simulink model "mobil_transporter"  (R2012b)
settings: Solver=FixedStepDiscrete  StartTime=0.0  StopTime=10.0  RelTol=1e-3
libraries: commutil2 x12, c2833xlib x8, c280xlib x6, idelinklib_tgtpref x2, simulink x1, idelinklib_ticcs x1
(part 1 of 2)
settings Model: Creator=User  LastModifiedBy=Gelin Wang
settings DataIOCC: SaveOutput=off  SaveTime=off
settings OptimizationCC: OptimizeModelRefInitCode=on  LifeSpan=1
settings HardwareCC: ProdBitPerChar=16  ProdBitPerInt=16  ProdBitPerPointer=16  ProdLargestAtomicInteger=Integer  ProdIntDivRoundTo=Zero  ProdEndianess=LittleEndian  ProdWordSize=16  ProdHWDeviceType=Texas Instruments->C2000
settings SFSimCC: SimCustomSourceCode="#include \"i2c_reset.c\""  SimCustomHeaderCode="#include \"i2c_reset.h\""
settings RTWCC: SystemTargetFile=idelink_ert.tlc  GenerateMakefile=off  TemplateMakefile=none  Description=IDE Link ERT  ProcessScript=idelink_ert_make_rtw_hook  RTWUseSimCustomCode=on  CustomSourceCode="#include \"i2c_reset.c\""  CustomHeaderCode="#include \"i2c_reset.h\""
settings CodeAppCC: IgnoreCustomStorageClasses=off

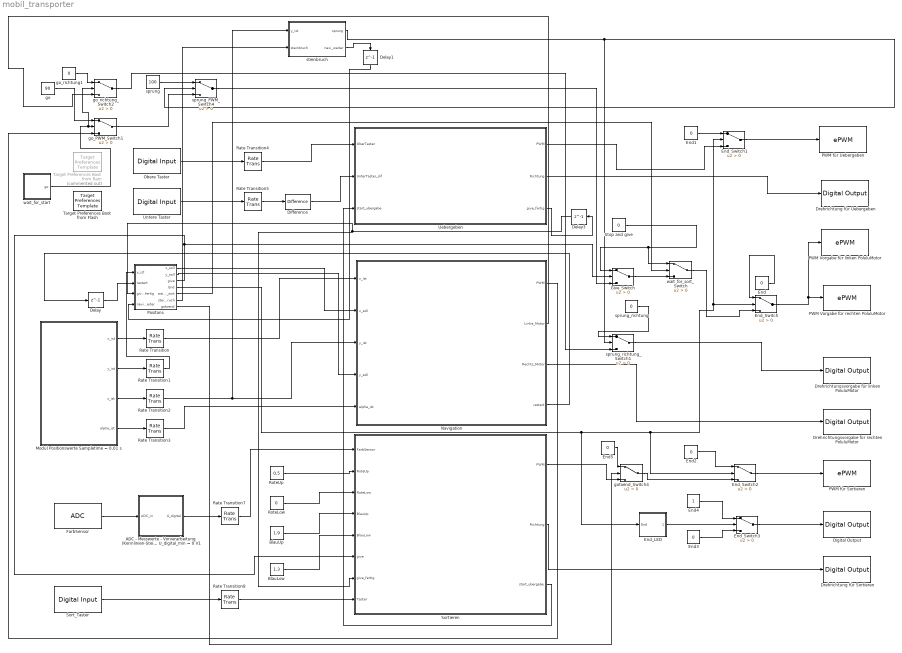
== system mobil_transporter ==
  "    go_PWM_Switch1" : Switch  Criteria=u2 > Threshold
  "    go_richtung_Switch2" : Switch  Criteria=u2 > Threshold
  "    sprung_PWM_Switch4" : Switch  Criteria=u2 > Threshold
  "    sprung_richtung_Switch1" : Switch  Criteria=u2 > Threshold
  ADC - Messwerte - Vorverarbeitung (Kennlinien-Steigung und Offset-Kompensation) U_digital = (ADC_in - Offset) * 3.546 V / 4096 mit U_digital_max = 3.546 V U_digital_min = 0 V1 : Subsystem
  BlauLow : Constant  Value=1.3
  BlauUp : Constant  Value=1.9
  Delay : Delay  DelayLength=1  InitialCondition=0
  Delay1 : Delay  DelayLength=1  InitialCondition=0
  Delay3 : Delay  DelayLength=1  InitialCondition=0
  Difference : simulink/Discrete/Difference  ICPrevInput=0.0  InputProcessing=Inherited  OutMin=[]  OutMax=[]  OutDataType=fixdt(1, 16)  OutScaling=2^-10  DoSatur=off
  Digital Output : c2833xlib/Digital Output  GPIO_Number=GPIO56~GPIO63  GPIO_Bit0=off  GPIO_BIT0_Toggle=off  GPIO_Bit1=off  GPIO_BIT1_Toggle=off  GPIO_Bit2=on  GPIO_BIT2_Toggle=off  GPIO_Bit3=off  GPIO_BIT3_Toggle=off  GPIO_Bit4=off  GPIO_BIT4_Toggle=off  GPIO_Bit5=off  GPIO_BIT5_Toggle=off  GPIO_Bit6=off  GPIO_BIT6_Toggle=off  GPIO_Bit7=off  GPIO_BIT7_Toggle=off
  Drehrichtung für Sortieren : c2833xlib/Digital Output  GPIO_Number=GPIO8~GPIO15  GPIO_Bit0=off  GPIO_BIT0_Toggle=off  GPIO_Bit1=off  GPIO_BIT1_Toggle=off  GPIO_Bit2=off  GPIO_BIT2_Toggle=off  GPIO_Bit3=off  GPIO_BIT3_Toggle=off  GPIO_Bit4=off  GPIO_BIT4_Toggle=off  GPIO_Bit5=off  GPIO_BIT5_Toggle=off  GPIO_Bit6=off  GPIO_BIT6_Toggle=off  GPIO_Bit7=on  GPIO_BIT7_Toggle=off
  Drehrichtung für Uebergeben : c2833xlib/Digital Output  GPIO_Number=GPIO16~GPIO23  GPIO_Bit0=on  GPIO_BIT0_Toggle=off  GPIO_Bit1=off  GPIO_BIT1_Toggle=off  GPIO_Bit2=off  GPIO_BIT2_Toggle=off  GPIO_Bit3=off  GPIO_BIT3_Toggle=off  GPIO_Bit4=off  GPIO_BIT4_Toggle=off  GPIO_Bit5=off  GPIO_BIT5_Toggle=off  GPIO_Bit6=off  GPIO_BIT6_Toggle=off  GPIO_Bit7=off  GPIO_BIT7_Toggle=off
  Drehrichtungsvorgabe für linken PoluluMotor : c2833xlib/Digital Output  GPIO_Number=GPIO16~GPIO23  GPIO_Bit0=off  GPIO_BIT0_Toggle=off  GPIO_Bit1=off  GPIO_BIT1_Toggle=off  GPIO_Bit2=off  GPIO_BIT2_Toggle=off  GPIO_Bit3=off  GPIO_BIT3_Toggle=off  GPIO_Bit4=off  GPIO_BIT4_Toggle=off  GPIO_Bit5=on  GPIO_BIT5_Toggle=off  GPIO_Bit6=off  GPIO_BIT6_Toggle=off  GPIO_Bit7=off  GPIO_BIT7_Toggle=off
  Drehrichtungsvorgabe für rechten PoluluMotor : c2833xlib/Digital Output  GPIO_Number=GPIO16~GPIO23  GPIO_Bit0=off  GPIO_BIT0_Toggle=off  GPIO_Bit1=off  GPIO_BIT1_Toggle=off  GPIO_Bit2=off  GPIO_BIT2_Toggle=off  GPIO_Bit3=off  GPIO_BIT3_Toggle=off  GPIO_Bit4=on  GPIO_BIT4_Toggle=off  GPIO_Bit5=off  GPIO_BIT5_Toggle=off  GPIO_Bit6=off  GPIO_BIT6_Toggle=off  GPIO_Bit7=off  GPIO_BIT7_Toggle=off
  End{,1..3,5} (5 alike) : Constant  Value=0
  End4 : Constant
  End_LED : Stateflow chart  TreatAsAtomicUnit=on
  End_Switch{,1..3} (4 alike) : Switch  Criteria=u2 > Threshold
  FarbSensor : c280xlib/ADC  useModule=A  useMode=Sequential  sourceSOC=Software  sourceSOC1=Software  sourceSOC2=ePWMxB  xint2_ADCSOC=31  Ts=0.001  dType=uint16  postInterrupt=off  numConversionsSingle=1  numConversionsDouble=1  conv0=ADCINA0  conv1=ADCINA1  conv2=ADCINA2  conv3=ADCINA3  conv4=ADCINA4  conv5=ADCINA5  conv6=ADCINA6  conv7=ADCINA7  conv8=ADCINB0  conv9=ADCINB1  conv10=ADCINB2  conv11=ADCINB3  conv12=ADCINB4  conv13=ADCINB5  conv14=ADCINB6  conv15=ADCINB7  convAB0=ADCINA0 and ADCINB0  convAB1=ADCINA1 and ADCINB1  convAB2=ADCINA2 and ADCINB2  convAB3=ADCINA3 and ADCINB3  convAB4=ADCINA4 and ADCINB4  convAB5=ADCINA5 and ADCINB5  convAB6=ADCINA6 and ADCINB6  convAB7=ADCINA7 and ADCINB7  convA0=ADCINA6  convA1=ADCINA2  convA2=ADCINA2  convA3=ADCINA3  convA4=ADCINA4  convA5=ADCINA5  convA6=ADCINA6  convA7=ADCINA7  convB0=ADCINB0  convB1=ADCINB1  convB2=ADCINB2  convB3=ADCINB3  convB4=ADCINB4  convB5=ADCINB5  convB6=ADCINB6  convB7=ADCINB7  c28xmultiPort=off  endma=off  chdma=1
  Give_Switch : Switch  Criteria=u2 > Threshold
  Modul Positionswerte Sampletime = 0.01 s : Subsystem
  Navigation : Subsystem
  Obere Taster : c2833xlib/Digital Input  GPIO_Number=GPIO24~GPIO31  GPIO_Bit0=on  GPIO_Bit1=off  GPIO_Bit2=off  GPIO_Bit3=off  GPIO_Bit4=off  GPIO_Bit5=off  GPIO_Bit6=off  GPIO_Bit7=off  sampleTime=0.01  dataType=auto  GPIO_Bit0_Qualification=Sync to SYSCLKOUT  GPIO_Bit1_Qualification=Sync to SYSCLKOUT  GPIO_Bit2_Qualification=Sync to SYSCLKOUT  GPIO_Bit3_Qualification=Sync to SYSCLKOUT  GPIO_Bit4_Qualification=Sync to SYSCLKOUT  GPIO_Bit5_Qualification=Sync to SYSCLKOUT  GPIO_Bit6_Qualification=Sync to SYSCLKOUT  GPIO_Bit7_Qualification=Sync to SYSCLKOUT  Qualification_Period=-1
  "PWM Vorgabe für linken PoluluMotor " : c280xlib/ePWM  checkMode=off  useModule=ePWM2  periodUnits=Clock cycles  timerSource=Specify via dialog  timerPeriod_clk=64000  timerPeriod_sec=0.0001  countingMode=Up  synchronizationOption=Disable  synchronizationEnable=off  phaseActiveEnable=Disable  phaseDirection=Count down after sync  phaseActive=0  clockPrescale=1  HSclockPrescale=1  ePWMxAStatus=off  CMPAUnits=Clock cycles  CMPASource=Specify via dialog  CMPAValue_per=50  CMPAValue_clk=32000  ePWMxAactionLogic1=Do nothing  ePWMxAactionLogic2=Clear  ePWMxAactionLogic3=Set  ePWMxAactionLogic4=Do nothing  ePWMxAactionLogic5=Do nothing  ePWMxAactionLogic6=Do nothing  ePWMxALoadMode=Load on CTR=Zero  ePWMxACSFenable=off  ePWMxACSFvalue=Forcing Disable  ePWMxASFreload=Zero  enHRPWM=off  HRPWM_LoadMode=CTR=ZERO  HRPWM_CTLMode=Phase control mode  HRPWM_EDGMode=Both edge  enSFO=on  ePWMxBStatus=on  CMPBUnits=Percentages  CMPBSource=Input port  CMPBValue_per=0  CMPBValue_clk=32000  ePWMxBactionLogic1=Do nothing  ePWMxBactionLogic2=Set  ePWMxBactionLogic3=Do nothing  ePWMxBactionLogic4=Do nothing  ePWMxBactionLogic5=Clear  ePWMxBactionLogic6=Do nothing  ePWMxBLoadMode=Load on CTR=Zero  ePWMxBCSFenable=off  ePWMxBCSFvalue=Forcing Disable  ePWMxBSFreload=Zero  enableDBePWMxA=off  enableDBePWMxB=off  DBpolarity=AH  DBedgeDelay=Positive  DBSource_ePWMxA=ePWMxA  DBSource_ePWMxB=ePWMxA  DBperiodSource=Specify via dialog  REDperiod=0  FEDperiod=0  adcstartModuleA=off  adcrequestEventA=First event  adcstartEventA=CTR=Zero  adcstartModuleB=off  adcrequestEventB=First event  adcstartEventB=CTR=Zero  intEn=off  intPrd=First event  intSel=CTR=Zero  chopperEnable=off  chopperFrequency=1  chopperFirstwidth=1  chopperDuty=12.5%  tripZonesource=Specify via dialog  tzselOSHT1=off  tzselOSHT2=off  tzselOSHT3=off  tzselOSHT4=off  tzselOSHT5=off  tzselOSHT6=off  tzselCBC1=off  tzselCBC2=off  tzselCBC3=off  tzselCBC4=off  tzselCBC5=off  tzselCBC6=off  enTzOstIntr=off  enTzCbcIntr=off  ePWMxAforced=No action  ePWMxBforced=No action  timerPeriod=-1  ePWMxAValue=0  ePWMxBValue=0  tripZoneoption=OSHT
  "PWM Vorgabe für rechten PoluluMotor " : c280xlib/ePWM  checkMode=off  useModule=ePWM1  periodUnits=Clock cycles  timerSource=Specify via dialog  timerPeriod_clk=64000  timerPeriod_sec=0.0001  countingMode=Up  synchronizationOption=Disable  synchronizationEnable=off  phaseActiveEnable=Disable  phaseDirection=Count down after sync  phaseActive=0  clockPrescale=1  HSclockPrescale=1  ePWMxAStatus=off  CMPAUnits=Clock cycles  CMPASource=Specify via dialog  CMPAValue_per=50  CMPAValue_clk=32000  ePWMxAactionLogic1=Do nothing  ePWMxAactionLogic2=Clear  ePWMxAactionLogic3=Set  ePWMxAactionLogic4=Do nothing  ePWMxAactionLogic5=Do nothing  ePWMxAactionLogic6=Do nothing  ePWMxALoadMode=Load on CTR=Zero  ePWMxACSFenable=off  ePWMxACSFvalue=Forcing Disable  ePWMxASFreload=Zero  enHRPWM=off  HRPWM_LoadMode=CTR=ZERO  HRPWM_CTLMode=Phase control mode  HRPWM_EDGMode=Both edge  enSFO=on  ePWMxBStatus=on  CMPBUnits=Percentages  CMPBSource=Input port  CMPBValue_per=0  CMPBValue_clk=32000  ePWMxBactionLogic1=Do nothing  ePWMxBactionLogic2=Set  ePWMxBactionLogic3=Do nothing  ePWMxBactionLogic4=Do nothing  ePWMxBactionLogic5=Clear  ePWMxBactionLogic6=Do nothing  ePWMxBLoadMode=Load on CTR=Zero  ePWMxBCSFenable=off  ePWMxBCSFvalue=Forcing Disable  ePWMxBSFreload=Zero  enableDBePWMxA=off  enableDBePWMxB=off  DBpolarity=AH  DBedgeDelay=Positive  DBSource_ePWMxA=ePWMxA  DBSource_ePWMxB=ePWMxA  DBperiodSource=Specify via dialog  REDperiod=0  FEDperiod=0  adcstartModuleA=off  adcrequestEventA=First event  adcstartEventA=CTR=Zero  adcstartModuleB=off  adcrequestEventB=First event  adcstartEventB=CTR=Zero  intEn=off  intPrd=First event  intSel=CTR=Zero  chopperEnable=off  chopperFrequency=1  chopperFirstwidth=1  chopperDuty=12.5%  tripZonesource=Specify via dialog  tzselOSHT1=off  tzselOSHT2=off  tzselOSHT3=off  tzselOSHT4=off  tzselOSHT5=off  tzselOSHT6=off  tzselCBC1=off  tzselCBC2=off  tzselCBC3=off  tzselCBC4=off  tzselCBC5=off  tzselCBC6=off  enTzOstIntr=off  enTzCbcIntr=off  ePWMxAforced=No action  ePWMxBforced=No action  timerPeriod=-1  ePWMxAValue=0  ePWMxBValue=0  tripZoneoption=OSHT
  PWM für Sortieren : c280xlib/ePWM  checkMode=off  useModule=ePWM5  periodUnits=Clock cycles  timerSource=Specify via dialog  timerPeriod_clk=64000  timerPeriod_sec=0.0001  countingMode=Up  synchronizationOption=Disable  synchronizationEnable=off  phaseActiveEnable=Disable  phaseDirection=Count down after sync  phaseActive=0  clockPrescale=1  HSclockPrescale=1  ePWMxAStatus=off  CMPAUnits=Clock cycles  CMPASource=Specify via dialog  CMPAValue_per=50  CMPAValue_clk=32000  ePWMxAactionLogic1=Do nothing  ePWMxAactionLogic2=Clear  ePWMxAactionLogic3=Set  ePWMxAactionLogic4=Do nothing  ePWMxAactionLogic5=Do nothing  ePWMxAactionLogic6=Do nothing  ePWMxALoadMode=Load on CTR=Zero  ePWMxACSFenable=off  ePWMxACSFvalue=Forcing Disable  ePWMxASFreload=Zero  enHRPWM=off  HRPWM_LoadMode=CTR=ZERO  HRPWM_CTLMode=Phase control mode  HRPWM_EDGMode=Both edge  enSFO=on  ePWMxBStatus=on  CMPBUnits=Percentages  CMPBSource=Input port  CMPBValue_per=0  CMPBValue_clk=32000  ePWMxBactionLogic1=Do nothing  ePWMxBactionLogic2=Set  ePWMxBactionLogic3=Do nothing  ePWMxBactionLogic4=Do nothing  ePWMxBactionLogic5=Clear  ePWMxBactionLogic6=Do nothing  ePWMxBLoadMode=Load on CTR=Zero  ePWMxBCSFenable=off  ePWMxBCSFvalue=Forcing Disable  ePWMxBSFreload=Zero  enableDBePWMxA=off  enableDBePWMxB=off  DBpolarity=AH  DBedgeDelay=Positive  DBSource_ePWMxA=ePWMxA  DBSource_ePWMxB=ePWMxA  DBperiodSource=Specify via dialog  REDperiod=0  FEDperiod=0  adcstartModuleA=off  adcrequestEventA=First event  adcstartEventA=CTR=Zero  adcstartModuleB=off  adcrequestEventB=First event  adcstartEventB=CTR=Zero  intEn=off  intPrd=First event  intSel=CTR=Zero  chopperEnable=off  chopperFrequency=1  chopperFirstwidth=1  chopperDuty=12.5%  tripZonesource=Specify via dialog  tzselOSHT1=off  tzselOSHT2=off  tzselOSHT3=off  tzselOSHT4=off  tzselOSHT5=off  tzselOSHT6=off  tzselCBC1=off  tzselCBC2=off  tzselCBC3=off  tzselCBC4=off  tzselCBC5=off  tzselCBC6=off  enTzOstIntr=off  enTzCbcIntr=off  ePWMxAforced=No action  ePWMxBforced=No action  timerPeriod=-1  ePWMxAValue=0  ePWMxBValue=0  tripZoneoption=OSHT
  PWM für Uebergeben : c280xlib/ePWM  checkMode=off  useModule=ePWM6  periodUnits=Clock cycles  timerSource=Specify via dialog  timerPeriod_clk=64000  timerPeriod_sec=0.0001  countingMode=Up  synchronizationOption=Disable  synchronizationEnable=off  phaseActiveEnable=Disable  phaseDirection=Count down after sync  phaseActive=0  clockPrescale=1  HSclockPrescale=1  ePWMxAStatus=off  CMPAUnits=Clock cycles  CMPASource=Specify via dialog  CMPAValue_per=50  CMPAValue_clk=32000  ePWMxAactionLogic1=Do nothing  ePWMxAactionLogic2=Clear  ePWMxAactionLogic3=Set  ePWMxAactionLogic4=Do nothing  ePWMxAactionLogic5=Do nothing  ePWMxAactionLogic6=Do nothing  ePWMxALoadMode=Load on CTR=Zero  ePWMxACSFenable=off  ePWMxACSFvalue=Forcing Disable  ePWMxASFreload=Zero  enHRPWM=off  HRPWM_LoadMode=CTR=ZERO  HRPWM_CTLMode=Phase control mode  HRPWM_EDGMode=Both edge  enSFO=on  ePWMxBStatus=on  CMPBUnits=Percentages  CMPBSource=Input port  CMPBValue_per=0  CMPBValue_clk=32000  ePWMxBactionLogic1=Do nothing  ePWMxBactionLogic2=Set  ePWMxBactionLogic3=Do nothing  ePWMxBactionLogic4=Do nothing  ePWMxBactionLogic5=Clear  ePWMxBactionLogic6=Do nothing  ePWMxBLoadMode=Load on CTR=Zero  ePWMxBCSFenable=off  ePWMxBCSFvalue=Forcing Disable  ePWMxBSFreload=Zero  enableDBePWMxA=off  enableDBePWMxB=off  DBpolarity=AH  DBedgeDelay=Positive  DBSource_ePWMxA=ePWMxA  DBSource_ePWMxB=ePWMxA  DBperiodSource=Specify via dialog  REDperiod=0  FEDperiod=0  adcstartModuleA=off  adcrequestEventA=First event  adcstartEventA=CTR=Zero  adcstartModuleB=off  adcrequestEventB=First event  adcstartEventB=CTR=Zero  intEn=off  intPrd=First event  intSel=CTR=Zero  chopperEnable=off  chopperFrequency=1  chopperFirstwidth=1  chopperDuty=12.5%  tripZonesource=Specify via dialog  tzselOSHT1=off  tzselOSHT2=off  tzselOSHT3=off  tzselOSHT4=off  tzselOSHT5=off  tzselOSHT6=off  tzselCBC1=off  tzselCBC2=off  tzselCBC3=off  tzselCBC4=off  tzselCBC5=off  tzselCBC6=off  enTzOstIntr=off  enTzCbcIntr=off  ePWMxAforced=No action  ePWMxBforced=No action  timerPeriod=-1  ePWMxAValue=0  ePWMxBValue=0  tripZoneoption=OSHT
  Positons : Stateflow chart  TreatAsAtomicUnit=on
  Rate Transition{,1..5,7..8} (8 alike) : RateTransition  OutPortSampleTime=0.01
  RoteLow : Constant  Value=0
  RoteUp : Constant  Value=0.5
  Sort_Taster : c2833xlib/Digital Input  GPIO_Number=GPIO24~GPIO31  GPIO_Bit0=off  GPIO_Bit1=off  GPIO_Bit2=on  GPIO_Bit3=off  GPIO_Bit4=off  GPIO_Bit5=off  GPIO_Bit6=off  GPIO_Bit7=off  sampleTime=0.01  dataType=auto  GPIO_Bit0_Qualification=Sync to SYSCLKOUT  GPIO_Bit1_Qualification=Sync to SYSCLKOUT  GPIO_Bit2_Qualification=Sync to SYSCLKOUT  GPIO_Bit3_Qualification=Sync to SYSCLKOUT  GPIO_Bit4_Qualification=Sync to SYSCLKOUT  GPIO_Bit5_Qualification=Sync to SYSCLKOUT  GPIO_Bit6_Qualification=Sync to SYSCLKOUT  GPIO_Bit7_Qualification=Sync to SYSCLKOUT  Qualification_Period=-1
  Sortieren : Subsystem
  Stop and give : Constant  Value=0
  Target Preferences Boot from Flash : idelinklib_tgtpref/Target Preferences Template  Tag=ccslinktgtpref_ccsv4  library=off
  Target Preferences Boot from Ram : idelinklib_tgtpref/Target Preferences Template  Tag=ccslinktgtpref_ccsv4  Commented=on  library=off
  Uebergeben : Stateflow chart  TreatAsAtomicUnit=on
  Untere Taster : c2833xlib/Digital Input  GPIO_Number=GPIO24~GPIO31  GPIO_Bit0=off  GPIO_Bit1=on  GPIO_Bit2=off  GPIO_Bit3=off  GPIO_Bit4=off  GPIO_Bit5=off  GPIO_Bit6=off  GPIO_Bit7=off  sampleTime=0.01  dataType=auto  GPIO_Bit0_Qualification=Sync to SYSCLKOUT  GPIO_Bit1_Qualification=Sync to SYSCLKOUT  GPIO_Bit2_Qualification=Sync to SYSCLKOUT  GPIO_Bit3_Qualification=Sync to SYSCLKOUT  GPIO_Bit4_Qualification=Sync to SYSCLKOUT  GPIO_Bit5_Qualification=Sync to SYSCLKOUT  GPIO_Bit6_Qualification=Sync to SYSCLKOUT  GPIO_Bit7_Qualification=Sync to SYSCLKOUT  Qualification_Period=-1
  go : Constant  Value=90
  go_richtung1 : Constant  Value=0
  gotoend_Switch4 : Switch  Criteria=u2 > Threshold
  sprung : Constant  Value=100
  sprung_richtung : Constant  Value=0
  steinbruch : Stateflow chart  TreatAsAtomicUnit=on
  wait_for_sort_Switch : Switch  Criteria=u2 > Threshold
  wait_for_start : Stateflow chart  TreatAsAtomicUnit=on
  wires:
  Modul Positionswerte Sampletime = 0.01 s/1(x_ist) -> Rate Transition/1
  Modul Positionswerte Sampletime = 0.01 s/4(alpha_ist) -> Rate Transition3/1
  Modul Positionswerte Sampletime = 0.01 s/3(z_ist) -> Rate Transition2/1
  Modul Positionswerte Sampletime = 0.01 s/2(y_ist) -> Rate Transition1/1
  Rate Transition/1 -> Navigation/1(x_ist)
  Delay/1 -> Positons/2(restart)
  Positons/3(give) -> Sortieren/6("give "), Give_Switch/2
  Stop and give/1 -> wait_for_sort_Switch/1, Give_Switch/1
  Rate Transition2/1 -> steinbruch/1(y_ist), Navigation/3(y_ist)
  Obere Taster/1 -> Rate Transition4/1
  Untere Taster/1 -> Rate Transition5/1
  Uebergeben/2(Richtung) -> Drehrichtung für Uebergeben/1
  Sortieren/2("Richtung ") -> Drehrichtung für Sortieren/1
  Positons/1(x_soll) -> Navigation/2(x_soll)
  Positons/2(y_soll) -> Navigation/4(y_soll)
  Navigation/3(Rechts_Motor) -> Drehrichtungsvorgabe für rechten PoluluMotor/1
  Navigation/4(restart) -> Delay/1
  Rate Transition3/1 -> Navigation/5(alpha_ist)
  Rate Transition4/1 -> Uebergeben/1(OberTaster)
  Rate Transition5/1 -> Difference/1
  Rate Transition7/1 -> Sortieren/1(FarbSensor)
  FarbSensor/1 -> ADC - Messwerte - Vorverarbeitung (Kennlinien-Steigung und Offset-Kompensation) U_digital = (ADC_in - Offset) * 3.546 V / 4096 mit U_digital_max = 3.546 V U_digital_min = 0 V1/1(ADC_in)
  ADC - Messwerte - Vorverarbeitung (Kennlinien-Steigung und Offset-Kompensation) U_digital = (ADC_in - Offset) * 3.546 V / 4096 mit U_digital_max = 3.546 V U_digital_min = 0 V1/1(U_digital) -> Rate Transition7/1
  Sort_Taster/1 -> Rate Transition8/1
  Rate Transition8/1 -> Sortieren/8(Taster)
  End/1 -> End_Switch/1
  Positons/4(End) -> End_LED/1(End), End_Switch2/2, End_Switch1/2, End_Switch/2
  Give_Switch/1 -> wait_for_sort_Switch/3
  End_Switch/1 -> "PWM Vorgabe für linken PoluluMotor "/1, "PWM Vorgabe für rechten PoluluMotor "/1
  End1/1 -> End_Switch1/1
  End_Switch1/1 -> PWM für Uebergeben/1
  End_Switch2/1 -> PWM für Sortieren/1
  Sortieren/1(PWM) -> gotoend_Switch4/3
  End2/1 -> End_Switch2/1
  Uebergeben/1(PWM) -> End_Switch1/3
  Difference/1 -> Uebergeben/2(UnterTaster_dif)
  Uebergeben/3(give_fertig) -> Delay3/1
  RoteUp/1 -> Sortieren/2(RoteUp)
  RoteLow/1 -> Sortieren/3(RoteLow)
  BlauUp/1 -> Sortieren/4(BlauUp)
  BlauLow/1 -> Sortieren/5(BlauLow)
  End_Switch3/1 -> Digital Output/1
  End3/1 -> End_Switch3/3
  End4/1 -> End_Switch3/1
  Sortieren/3(start_ubergabe) -> Uebergeben/3(start_ubergabe)
  Delay3/1 -> Sortieren/7(give_fertig), Positons/3(give_fertig)
  Positons/5(wait_for_sort) -> wait_for_sort_Switch/2
  wait_for_sort_Switch/1 -> End_Switch/3
  sprung/1 -> "    sprung_PWM_Switch4"/1
  "    sprung_PWM_Switch4"/1 -> Give_Switch/3
  sprung_richtung/1 -> "    sprung_richtung_Switch1"/1
  "    sprung_richtung_Switch1"/1 -> Drehrichtungsvorgabe für linken PoluluMotor/1
  wait_for_start/1(go) -> "    go_richtung_Switch2"/2, "    go_PWM_Switch1"/2
  go/1 -> "    go_PWM_Switch1"/1
  "    go_PWM_Switch1"/1 -> "    sprung_PWM_Switch4"/3
  Navigation/1(PWM) -> "    go_PWM_Switch1"/3
  Rate Transition1/1 -> Positons/1(y_ist)
  "    go_richtung_Switch2"/1 -> "    sprung_richtung_Switch1"/3
  go_richtung1/1 -> "    go_richtung_Switch2"/1
  Navigation/2(Linke_Motor) -> "    go_richtung_Switch2"/3
  steinbruch/1(sprung) -> "    sprung_richtung_Switch1"/2, "    sprung_PWM_Switch4"/2
  Positons/6(steinbruch) -> steinbruch/2(steinbruch)
  steinbruch/2(navi_weiter) -> Delay1/1
  Delay1/1 -> Positons/4(navi_weiter)
  End5/1 -> gotoend_Switch4/1
  gotoend_Switch4/1 -> End_Switch2/3
  Positons/7(gotoend) -> gotoend_Switch4/2
  End_LED/1(End_now) -> End_Switch3/2

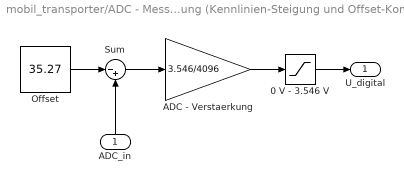
== system mobil_transporter/ADC - Messwerte - Vorverarbeitung (Kennlinien-Steigung und Offset-Kompensation) U_digital = (ADC_in - Offset) * 3.546 V // 4096 mit U_digital_max = 3.546 V U_digital_min = 0 V1 ==
  ADC_in : Inport
  0 V - 3.546 V : Saturate  UpperLimit=3.546  LowerLimit=0
  ADC - Verstaerkung : Gain  Gain=3.546/4096
  Offset : Constant  Value=35.27
  Sum : Sum  Inputs=|-+
  U_digital : Outport
  wires:
  ADC - Verstaerkung/1 -> 0 V - 3.546 V/1
  Sum/1 -> ADC - Verstaerkung/1
  Offset/1 -> Sum/1
  0 V - 3.546 V/1 -> U_digital/1
  ADC_in/1 -> Sum/2

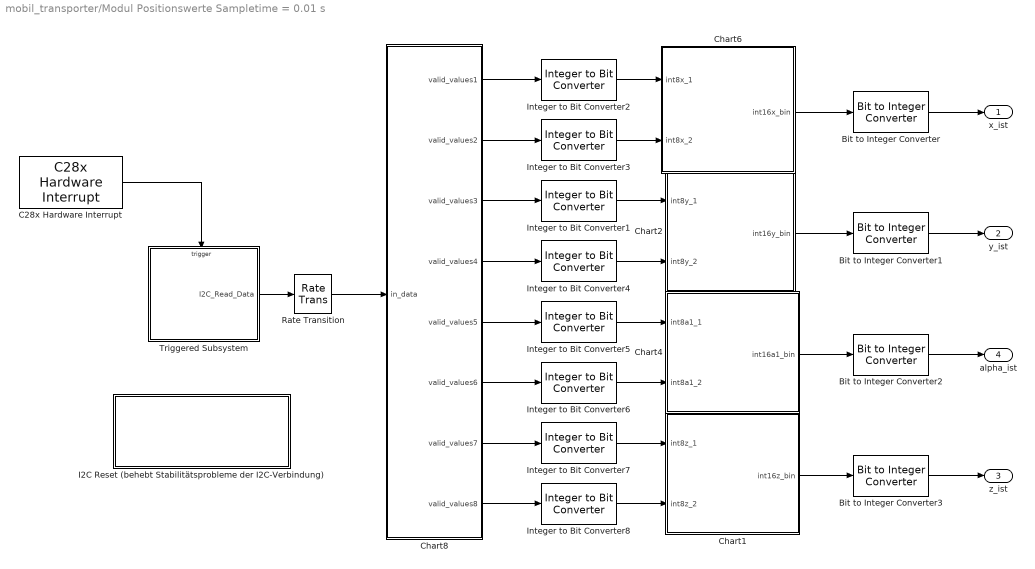
== system mobil_transporter/Modul Positionswerte Sampletime = 0.01 s ==
  Bit to Integer Converter{,1..3} (4 alike) : commutil2/Bit to Integer Converter  nbits=16  bitOrder=MSB first  signedOutputValues=Signed  outDtype=Inherit via internal rule  outDtypeSigned=Inherit via internal rule
  C28x Hardware Interrupt : idelinklib_ticcs/C28x Hardware Interrupt  irqnumbers=8  pienumbers=2  irqpriorities=30  irqpreempts=0  showinput=off  dspchiptype=C280X
  Chart1 : Stateflow chart  TreatAsAtomicUnit=on
  Chart2 : Stateflow chart  TreatAsAtomicUnit=on
  Chart4 : Stateflow chart  TreatAsAtomicUnit=on
  Chart6 : Stateflow chart  TreatAsAtomicUnit=on
  Chart8 : Stateflow chart  TreatAsAtomicUnit=on
  I2C Reset (behebt Stabilitätsprobleme der I2C-Verbindung) : Subsystem
  Integer to Bit Converter{1..8} (8 alike) : commutil2/Integer to Bit Converter  nbits=8  signedInputValues=Unsigned  bitOrder=MSB first  outDtype=uint8
  Rate Transition : RateTransition  Deterministic=off  OutPortSampleTime=0.01
  Triggered Subsystem : Subsystem  TreatAsAtomicUnit=on
  x_ist : Outport
  y_ist : Outport  Port=2
  z_ist : Outport  Port=3
  alpha_ist : Outport  Port=4
  wires:
  Integer to Bit Converter7/1 -> Chart1/1(int8z_1)
  Integer to Bit Converter8/1 -> Chart1/2(int8z_2)
  Chart8/7(valid_values7) -> Integer to Bit Converter7/1
  Chart8/8(valid_values8) -> Integer to Bit Converter8/1
  Bit to Integer Converter3/1 -> z_ist/1
  Triggered Subsystem/1(I2C_Read_Data) -> Rate Transition/1
  Chart1/1(int16z_bin) -> Bit to Integer Converter3/1
  Chart4/1(int16a1_bin) -> Bit to Integer Converter2/1
  Chart8/6(valid_values6) -> Integer to Bit Converter6/1
  Bit to Integer Converter2/1 -> alpha_ist/1
  Bit to Integer Converter/1 -> x_ist/1
  Integer to Bit Converter6/1 -> Chart4/2(int8a1_2)
  Integer to Bit Converter5/1 -> Chart4/1(int8a1_1)
  Integer to Bit Converter4/1 -> Chart2/2(int8y_2)
  Integer to Bit Converter2/1 -> Chart6/1(int8x_1)
  Integer to Bit Converter1/1 -> Chart2/1(int8y_1)
  Chart6/1(int16x_bin) -> Bit to Integer Converter/1
  Integer to Bit Converter3/1 -> Chart6/2(int8x_2)
  Chart8/3(valid_values3) -> Integer to Bit Converter1/1
  Chart8/1(valid_values1) -> Integer to Bit Converter2/1
  Chart2/1(int16y_bin) -> Bit to Integer Converter1/1
  Chart8/4(valid_values4) -> Integer to Bit Converter4/1
  Chart8/2(valid_values2) -> Integer to Bit Converter3/1
  Chart8/5(valid_values5) -> Integer to Bit Converter5/1
  C28x Hardware Interrupt/1 -> Triggered Subsystem/Trigger
  Rate Transition/1 -> Chart8/1(in_data)
  Bit to Integer Converter1/1 -> y_ist/1

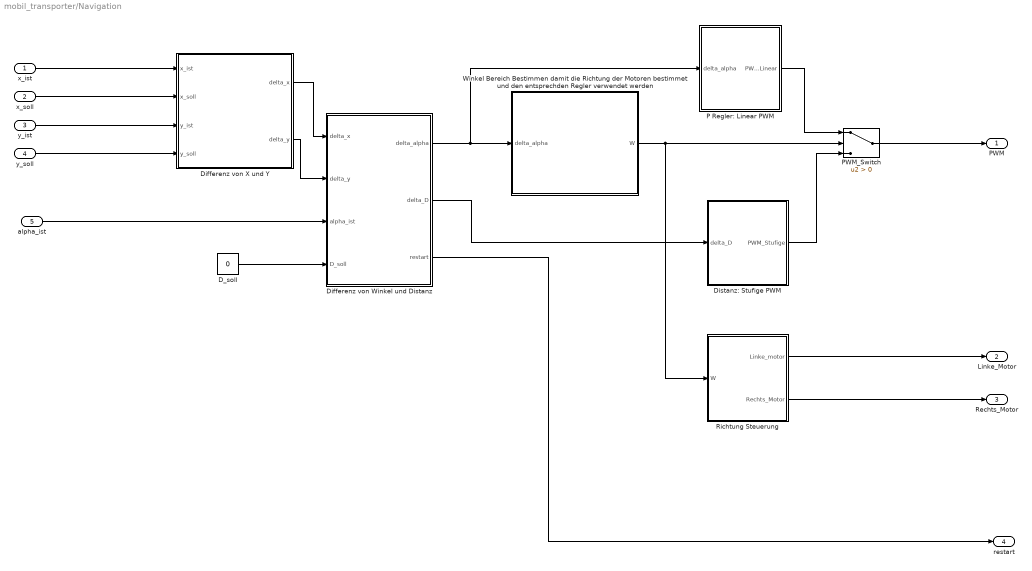
== system mobil_transporter/Navigation ==
  x_ist : Inport
  x_soll : Inport  Port=2
  y_ist : Inport  Port=3
  y_soll : Inport  Port=4
  alpha_ist : Inport  Port=5
  D_soll : Constant  Value=0
  Differenz von Winkel und Distanz : Subsystem
  Differenz von X und Y : Subsystem
  Distanz: Stufige PWM : Subsystem
  P Regler: Linear PWM : Subsystem
  PWM_Switch : Switch  Criteria=u2 > Threshold
  Richtung Steuerung : Subsystem
  Winkel Bereich Bestimmen damit die Richtung der Motoren bestimmet und den entsprechden Regler verwendet werden : Subsystem
  PWM : Outport
  Linke_Motor : Outport  Port=2
  Rechts_Motor : Outport  Port=3
  restart : Outport  Port=4
  wires:
  Differenz von Winkel und Distanz/1(delta_alpha) -> P Regler: Linear PWM/1(delta_alpha), Winkel Bereich Bestimmen damit die Richtung der Motoren bestimmet und den entsprechden Regler verwendet werden/1(delta_alpha)
  Winkel Bereich Bestimmen damit die Richtung der Motoren bestimmet und den entsprechden Regler verwendet werden/1(W) -> Richtung Steuerung/1(W), PWM_Switch/2
  P Regler: Linear PWM/1(PWM_Linear) -> PWM_Switch/1
  Distanz: Stufige PWM/1(PWM_Stufige) -> PWM_Switch/3
  Richtung Steuerung/1(Linke_motor) -> Linke_Motor/1
  Richtung Steuerung/2(Rechts_Motor) -> Rechts_Motor/1
  Differenz von X und Y/1(delta_x) -> Differenz von Winkel und Distanz/1(delta_x)
  Differenz von X und Y/2(delta_y) -> Differenz von Winkel und Distanz/2(delta_y)
  alpha_ist/1 -> Differenz von Winkel und Distanz/3(alpha_ist)
  D_soll/1 -> Differenz von Winkel und Distanz/4(D_soll)
  Differenz von Winkel und Distanz/2(delta_D) -> Distanz: Stufige PWM/1(delta_D)
  Differenz von Winkel und Distanz/3(restart) -> restart/1
  PWM_Switch/1 -> PWM/1
  x_ist/1 -> Differenz von X und Y/1(x_ist)
  x_soll/1 -> Differenz von X und Y/2(x_soll)
  y_ist/1 -> Differenz von X und Y/3(y_ist)
  y_soll/1 -> Differenz von X und Y/4(y_soll)

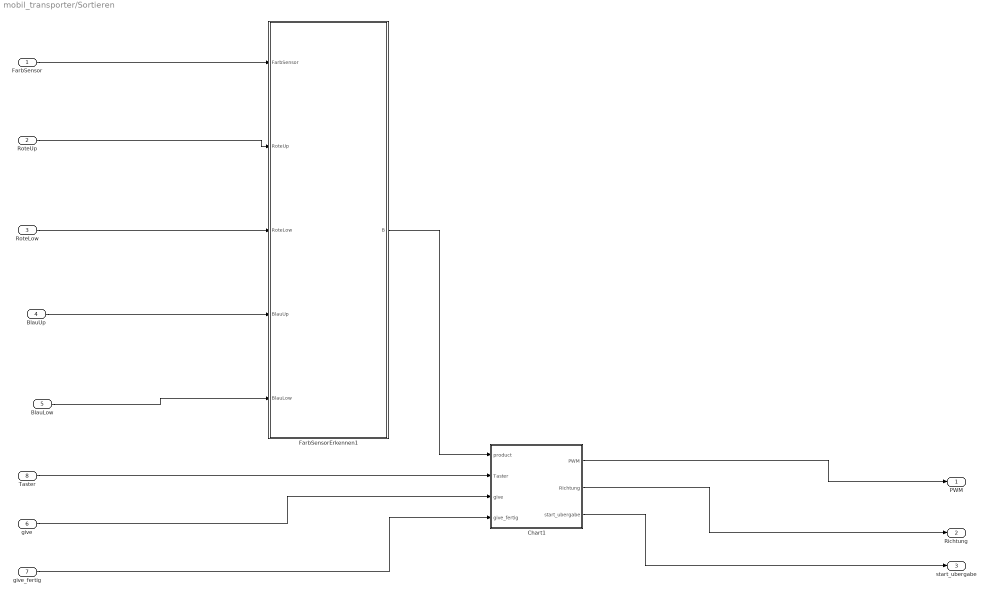
== system mobil_transporter/Sortieren ==
  FarbSensor : Inport
  RoteUp : Inport  Port=2
  RoteLow : Inport  Port=3
  BlauUp : Inport  Port=4
  BlauLow : Inport  Port=5
  "give " : Inport  Port=6
  give_fertig : Inport  Port=7
  Taster : Inport  Port=8
  Chart1 : Stateflow chart  TreatAsAtomicUnit=on
  FarbSensorErkennen1 : MATLAB Function  TreatAsAtomicUnit=on
  PWM : Outport
  "Richtung " : Outport  Port=2
  start_ubergabe : Outport  Port=3
  wires:
  Chart1/2(Richtung) -> "Richtung "/1
  Taster/1 -> Chart1/2(Taster)
  Chart1/1(PWM) -> PWM/1
  FarbSensorErkennen1/1(B) -> Chart1/1(product)
  FarbSensor/1 -> FarbSensorErkennen1/1(FarbSensor)
  RoteUp/1 -> FarbSensorErkennen1/2(RoteUp)
  RoteLow/1 -> FarbSensorErkennen1/3(RoteLow)
  BlauUp/1 -> FarbSensorErkennen1/4(BlauUp)
  BlauLow/1 -> FarbSensorErkennen1/5(BlauLow)
  "give "/1 -> Chart1/3(give)
  Chart1/3(start_ubergabe) -> start_ubergabe/1
  give_fertig/1 -> Chart1/4(give_fertig)

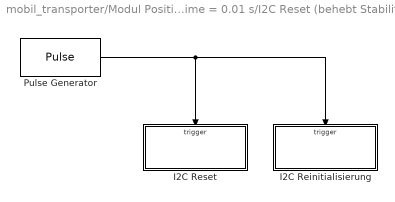
== system mobil_transporter/Modul Positionswerte Sampletime = 0.01 s/I2C Reset (behebt Stabilitätsprobleme der I2C-Verbindung) ==
  I2C Reinitialisierung : Subsystem  TreatAsAtomicUnit=on
  I2C Reset : Subsystem  TreatAsAtomicUnit=on
  Pulse Generator : DiscretePulseGenerator  Period=250  SampleTime=0.01
  wires:
  Pulse Generator/1 -> I2C Reset/Trigger, I2C Reinitialisierung/Trigger

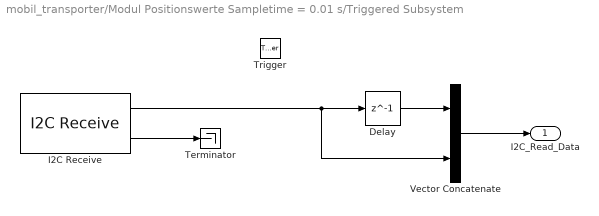
== system mobil_transporter/Modul Positionswerte Sampletime = 0.01 s/Triggered Subsystem ==
  Trigger : TriggerPort  TriggerType=function-call
  Delay : Delay  DelayLength=1  InitialCondition=0
  I2C Receive : c280xlib/I2C Receive  addrFormat=7-Bit addressing  saSource=Specify via dialog  SAR=80  bitCount=8  dataLength=10  initValue=0  NACK=on  STP=off  STR=on  sampleTime=-1  dataType=uint8
  Terminator : Terminator
  Vector Concatenate : Concatenate
  I2C_Read_Data : Outport
  wires:
  I2C Receive/2 -> Terminator/1
  I2C Receive/1 -> Vector Concatenate/2, Delay/1
  Delay/1 -> Vector Concatenate/1
  Vector Concatenate/1 -> I2C_Read_Data/1

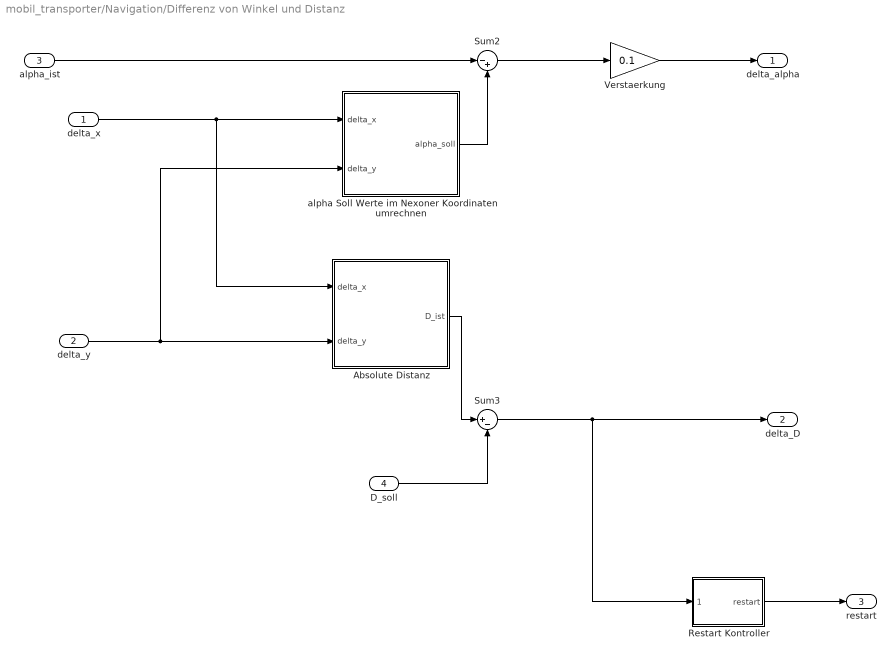
== system mobil_transporter/Navigation/Differenz von Winkel und Distanz ==
  delta_x : Inport
  delta_y : Inport  Port=2
  alpha_ist : Inport  Port=3
  D_soll : Inport  Port=4
  Absolute Distanz : MATLAB Function  TreatAsAtomicUnit=on  SystemSampleTime=0.01
  Restart Kontroller : MATLAB Function  TreatAsAtomicUnit=on
  Sum2 : Sum  Inputs=|-+  SampleTime=0.01
  Sum3 : Sum  Inputs=|+-  SampleTime=0.01
  Verstaerkung : Gain  Gain=0.1  SampleTime=0.01
  alpha Soll Werte im Nexoner Koordinaten umrechnen : MATLAB Function  TreatAsAtomicUnit=on  SystemSampleTime=0.01
  delta_alpha : Outport
  delta_D : Outport  Port=2
  restart : Outport  Port=3
  wires:
  alpha Soll Werte im Nexoner Koordinaten umrechnen/1(alpha_soll) -> Sum2/2
  alpha_ist/1 -> Sum2/1
  Sum2/1 -> Verstaerkung/1
  Sum3/1 -> delta_D/1, Restart Kontroller/1(delta_D)
  D_soll/1 -> Sum3/2
  Absolute Distanz/1(D_ist) -> Sum3/1
  Verstaerkung/1 -> delta_alpha/1
  delta_x/1 -> Absolute Distanz/1(delta_x), alpha Soll Werte im Nexoner Koordinaten umrechnen/1(delta_x)
  delta_y/1 -> Absolute Distanz/2(delta_y), alpha Soll Werte im Nexoner Koordinaten umrechnen/2(delta_y)
  Restart Kontroller/1(restart) -> restart/1

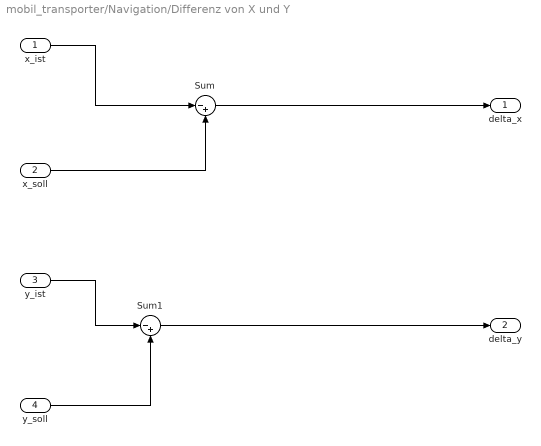
== system mobil_transporter/Navigation/Differenz von X und Y ==
  x_ist : Inport
  x_soll : Inport  Port=2
  y_ist : Inport  Port=3
  y_soll : Inport  Port=4
  Sum : Sum  Inputs=|-+
  Sum1 : Sum  Inputs=|-+
  delta_x : Outport
  delta_y : Outport  Port=2
  wires:
  x_ist/1 -> Sum/1
  x_soll/1 -> Sum/2
  y_ist/1 -> Sum1/1
  y_soll/1 -> Sum1/2
  Sum/1 -> delta_x/1
  Sum1/1 -> delta_y/1

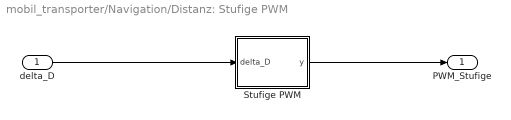
== system mobil_transporter/Navigation/Distanz: Stufige PWM ==
  delta_D : Inport
  "Stufige PWM " : MATLAB Function  TreatAsAtomicUnit=on
  PWM_Stufige : Outport
  wires:
  delta_D/1 -> "Stufige PWM "/1(delta_D)
  "Stufige PWM "/1(y) -> PWM_Stufige/1

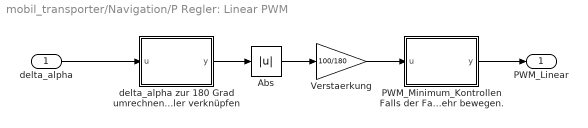
== system mobil_transporter/Navigation/P Regler: Linear PWM ==
  delta_alpha : Inport
  Abs : Abs
  "PWM_Minimum_Kontrollen Falls der Fahrzeug zu schwer ist, kann es sich nicht mehr bewegen. " : MATLAB Function  TreatAsAtomicUnit=on
  Verstaerkung : Gain  Gain=100/180  SampleTime=0.01
  delta_alpha zur 180 Grad umrechnen damit es mit P Regler verknüpfen : MATLAB Function  TreatAsAtomicUnit=on
  PWM_Linear : Outport
  wires:
  delta_alpha/1 -> delta_alpha zur 180 Grad umrechnen damit es mit P Regler verknüpfen/1(u)
  Verstaerkung/1 -> "PWM_Minimum_Kontrollen Falls der Fahrzeug zu schwer ist, kann es sich nicht mehr bewegen. "/1(u)
  delta_alpha zur 180 Grad umrechnen damit es mit P Regler verknüpfen/1(y) -> Abs/1
  Abs/1 -> Verstaerkung/1
  "PWM_Minimum_Kontrollen Falls der Fahrzeug zu schwer ist, kann es sich nicht mehr bewegen. "/1(y) -> PWM_Linear/1

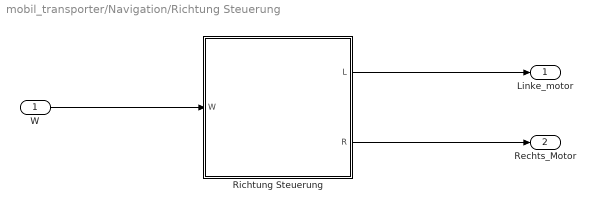
== system mobil_transporter/Navigation/Richtung Steuerung ==
  W : Inport
  Richtung Steuerung : MATLAB Function  TreatAsAtomicUnit=on
  Linke_motor : Outport
  Rechts_Motor : Outport  Port=2
  wires:
  Richtung Steuerung/2(R) -> Rechts_Motor/1
  Richtung Steuerung/1(L) -> Linke_motor/1
  W/1 -> Richtung Steuerung/1(W)

== system mobil_transporter/Navigation/Winkel Bereich Bestimmen damit die Richtung der Motoren bestimmet und den entsprechden Regler verwendet werden ==
  delta_alpha : Inport
  WinkelVergleich : MATLAB Function  TreatAsAtomicUnit=on  SystemSampleTime=0.01
  W : Outport
  wires:
  delta_alpha/1 -> WinkelVergleich/1(u)
  WinkelVergleich/1(W) -> W/1

== system mobil_transporter/Modul Positionswerte Sampletime = 0.01 s/I2C Reset (behebt Stabilitätsprobleme der I2C-Verbindung)/I2C Reinitialisierung ==
  Trigger : TriggerPort  TriggerType=falling
  I2C Reinitialisierung : MATLAB Function  TreatAsAtomicUnit=on

== system mobil_transporter/Modul Positionswerte Sampletime = 0.01 s/I2C Reset (behebt Stabilitätsprobleme der I2C-Verbindung)/I2C Reset ==
  Trigger : TriggerPort
  I2C Reset : MATLAB Function  TreatAsAtomicUnit=on

== stateflow chart mobil_transporter/wait_for_start ==
  state wait
    en:go=1;
  state Go
    en:go=0;
  (default) -> wait
  wait -> Go : after(3.5,sec)
  data: go output

== stateflow chart mobil_transporter/steinbruch ==
  state vordecide
    en:navi_weiter=0;
  state sprung
    en:sprung=1;
  state navi_weiter
    en:navi_weiter=1;
    en:sprung=0;
  (default) -> vordecide
  navi_weiter -> vordecide : after(0.1,sec)
  vordecide -> sprung : [steinbruch==1]
  sprung -> navi_weiter : after(0.7,sec)
  data: y_ist input; sprung output; y_now_1 local double; y_now_2 local double; steinbruch input; navi_weiter output double

== stateflow chart mobil_transporter/End_LED ==
  state LED_on_1
    en:End_now=1;
  state Start_to_count
  state LED_on_2
    en:End_now=1;
  (default) -> Start_to_count
  Start_to_count -> LED_on_1 [order 2] : [End==1]
  Start_to_count -> LED_on_2 [order 1] : after(175,sec)
  data: End input double =0; End_now output double =0

== matlab function mobil_transporter/Navigation/Differenz von Winkel und Distanz/Absolute Distanz ==
  settings: updateMethod=DISCRETE  sampleTime=0.01
  data: delta_x input; D_ist output; delta_y input
function D_ist = fcn( delta_x,delta_y )

%%Absolute Distanz zwischen aktuelle Stelle und Ziel

D_ist = sqrt((delta_x)^2 + (delta_y)^2);

end

== matlab function mobil_transporter/Navigation/Richtung Steuerung/Richtung Steuerung ==
  data: W input; L output; R output
function [L,R] = fcn(W)
if W == 1
    %%Links Abbiegen
    L = 1;
    R = 1;
elseif W == 2
    %%Rechts Abbiegen
    L = 0;
    R = 0;
else
    %%Gerade Fahren
    L = 0;
    R = 1;
end

== stateflow chart mobil_transporter/Positons ==
  state Position_6
    en:x_soll=9000;
    en:y_soll=8000;
  state Position_7
    en:x_soll=9600;
    en:y_soll=6600;
  state Position_8
    en:x_soll=10000;
    en:y_soll=6100;
  state Position_5
    en:x_soll=8500;
    en:y_soll=2500;
  state Position_1
  state Position_2
    en:x_soll=2200;
    en:y_soll=7000;
  state Position_3
    en:x_soll=4900;
    en:y_soll=9200;
  state Position_4
    en:x_soll=6700;
    en:y_soll=7500;
  state Position_9
    en:x_soll=12000;
    en:y_soll=4500;
  state Stop_and_Give_1
    en:give=1;
    en:wait_for_sort=0;
  state Position_10
    en:give=0;
    en:x_soll=10800;
    en:y_soll=950;
  state wait_for_sort
    en:wait_for_sort=1;
  state Position_11
    en:x_soll=14000;
    en:y_soll=950;
  state Position_Give_1
    en:x_soll=10200;
    en:y_soll=1150;
  state steckt2
    en:steinbruch=1;
    exit:steinbruch=0;
  state Position_16
    en:x_soll=14000;
    en:y_soll=9100;
  state Position_18
    en:x_soll=8000;
    en:y_soll=8500;
  state Positon_14
    en:x_soll=17000;
    en:y_soll=9350
  state Position_17
    en:x_soll=12000;
    en:y_soll=9200;
  state Position_15
    en:x_soll=15000;
    en:y_soll=8980;
  state Position_12
    en:x_soll=17500;
    en:y_soll=2000;
  state Position_13
    en:x_soll=17400;
    en:y_soll=4000;
  state steckt3
    en:steinbruch=1;
    exit:steinbruch=0;
  state steckt1
    en:steinbruch=1;
    exit:steinbruch=0;
  state steckt
    en:steinbruch=1;
    exit:steinbruch=0;
  state Position_19
    en:x_soll=6000;
    en:y_soll=7000;
  state wait_for_sort1
    en:wait_for_sort=1;
  state Position_Give_2
    en:x_soll=10500;
    en:y_soll=1150;
  state Position_20
    en:x_soll=9600;
    en:y_soll=6600;
  state Stop_and_Give_2
    en:give=1;
    en:wait_for_sort=0;
  state Position_22
    en:x_soll=10500;
    en:y_soll=4500;
  state Position_21
    en:x_soll=10000;
    en:y_soll=6100;
  state Position_23
    en:give=0;
    en:gotoend=1;
    en:x_soll=11000;
    en:y_soll=100;
  state Position_25
    en:x_soll=10500;
    en:y_soll=-1250;
  state Position_24
    en:x_soll=7000;
    en:y_soll=0;
  state Stop
    en:End=1;
  state steckt4
    en:steinbruch=1;
    exit:steinbruch=0;
  (default) -> Position_1
  Position_6 -> Position_7 : [restart==1]
  Position_7 -> Position_8 : [restart==1]
  Position_5 -> Position_6 : [restart==1]
  Position_3 -> Position_4 : [restart==1]
  Position_2 -> Position_3 : [restart==1]
  Position_4 -> Position_5 : [restart==1]
  Position_8 -> Position_9 : [restart==1]
  Position_1 -> Position_2 : [restart==1]
  Position_9 -> Position_Give_1
  wait_for_sort -> Stop_and_Give_1 : after(16,sec)
  Stop_and_Give_1 -> Position_10 : [give_fertig==1]
  Position_Give_1 -> wait_for_sort : [restart==1]
  Position_10 -> Position_11 : [restart==1]
  steckt2 -> Position_18 : [navi_weiter==1]
  Position_11 -> Position_12 : [restart==1]
  Position_18 -> steckt2 [order 1] : after(5,sec)
  steckt1 -> Position_15 : [navi_weiter==1]
  Position_17 -> Position_18 : [restart==1]
  Position_12 -> Position_13 : [restart==1]
  Position_16 -> Position_17 [order 2] : [restart==1]
  Positon_14 -> Position_15 [order 2] : [restart==1]
  Position_15 -> Position_16 [order 2] : [restart==1]
  Position_13 -> Positon_14 : [restart==1]
  steckt3 -> Position_16 : [navi_weiter==1]
  steckt -> Positon_14 : [navi_weiter==1]
  Position_15 -> steckt1 [order 1] : after(4,sec)
  Position_18 -> Position_19 [order 2] : [restart==1]
  Positon_14 -> steckt [order 1] : after(4,sec)
  Position_16 -> steckt3 [order 1] : after(4,sec)
  Position_Give_2 -> wait_for_sort1 : [restart==1]
  Position_23 -> steckt4 [order 1] : after(5,sec)
  Position_21 -> Position_22 : [restart==1]
  Position_20 -> Position_21 : [restart==1]
  Position_22 -> Position_Give_2 : [restart==1]
  steckt4 -> Position_23 : [navi_weiter==1]
  wait_for_sort1 -> Stop_and_Give_2 : after(7,sec)
  Stop_and_Give_2 -> Position_23 : [give_fertig==1]
  Position_19 -> Position_20 : [restart==1]
  Position_23 -> Position_24 [order 2] : [restart==1]
  Position_24 -> Position_25 : [restart==1]
  Position_25 -> Stop : [restart==1]
  data: x_soll output double =3500; y_soll output double =2500; y_ist input double; restart input double; give output double =0; End output double =0; give_fertig input double; wait_for_sort output double =0; steinbruch output double =0; navi_weiter input; gotoend output double =0

== stateflow chart mobil_transporter/Sortieren/Chart1 ==
  state give_decide
    en:PWM=0;
    en:start_ubergabe=0;
  state Initializierung
    en:c=0;
  state AufTaster_1
  state Drehen
    en:PWM=50;
    en:Richtung=0;
  state decide
  state Start
    en:PWM=0;
  state AufTaster
  state Collision
    en:PWM=50,
    en:Richtung=0;
    exit:letzteRichtung=0;
  state Pause
    en:temp=0;
  state Logik
    en:temp=product;
  state AufTaster_2
  state Rote
    en:PWM=50;
    en: Richtung=0;
    exit: letzteRichtung = 0;
  state Blau
    en:PWM=50;
    en: Richtung=1;
    exit: letzteRichtung = 1;
  state sicherheit
    en:PWM=50;
    en:Richtung = (letzteRichtung-1)*(-1);
    exit:c=c+1;
    exit:letzteRichtung=Richtung;
  state No_collision
    en:PWM=0;
    en:start_ubergabe=1;
  state reset_Muell
    en:c=0;
    en:PWM=60;
  state ignorieren
  (default) -> give_decide
  give_decide -> Initializierung [order 2] : [give==0]
  No_collision -> give_decide : [give_fertig==1]
  give_decide -> decide [order 1] : [give==1]
  AufTaster -> give_decide : [Taster==0]
  Initializierung -> Start : [c==0]
  Drehen -> AufTaster : [Taster==1]
  AufTaster_1 -> Drehen [order 1] : [product==temp]
  AufTaster_1 -> Pause [order 2] : [product != 2]
  Logik -> AufTaster_1 [order 1] : after(2,sec)
  decide -> No_collision [order 1] : [letzteRichtung==0]
  decide -> Collision [order 2] : [letzteRichtung==1]
  Start -> Pause : after(1,sec)
  ignorieren -> AufTaster : [Taster ==1 ]
  sicherheit -> AufTaster [order 2] : [Taster==1]
  Rote -> AufTaster [order 2] : [Taster ==1 && letzteRichtung == 0]
  Blau -> AufTaster [order 2] : [Taster ==1 && letzteRichtung == 1]
  Logik -> Pause [order 2] : [product != 2]
  Pause -> Logik [order 2] : [product==2]
  Pause -> Rote [order 3] : [ product == 0 ]
  Pause -> Blau [order 1] : [ product == 1 ]
  Collision -> AufTaster_2 : [Taster==1]
  AufTaster_2 -> No_collision : [Taster==0]
  Rote -> ignorieren [order 1] : [Taster ==1 && letzteRichtung == 1]
  Rote -> sicherheit [order 3] : after(3,sec)
  Blau -> sicherheit [order 3] : after(3,sec)
  Blau -> ignorieren [order 1] : [Taster ==1 && letzteRichtung == 0]
  sicherheit -> reset_Muell [order 1] : [c==4]
  reset_Muell -> ignorieren : [Taster==1]
  data: product input; Taster input; PWM output; Richtung output =0; letzteRichtung local double =0; temp local double; c local double; give input; start_ubergabe output double; give_fertig input

== matlab function mobil_transporter/Sortieren/FarbSensorErkennen1 ==
  data: FarbSensor input; B output; RoteUp input; RoteLow input; BlauUp input; BlauLow input
function B = fcn(FarbSensor,RoteUp,RoteLow,BlauUp,BlauLow)
if FarbSensor <= RoteUp && FarbSensor >= RoteLow 
    %%Rote Stein
    B = 0;
elseif FarbSensor < BlauUp && FarbSensor >= BlauLow
    %%Blaue Stein
    B = 1;
else
    %%Keinen Stein kommt oder Schwarz
    B = 2;
end

== stateflow chart mobil_transporter/Modul Positionswerte Sampletime = 0.01 s/Chart1 ==
  state Daten_einlesen
  state x0
  state x1_1
    int16z_bin[0] = int8z_1[0];
    int16z_bin[1] = int8z_1[1];
    int16z_bin[2] = int8z_1[2];
    int16z_bin[3] = int8z_1[3];
    int16z_bin[4] = int8z_1[4];
    int16z_bin[5] = int8z_1[5]
    int16z_bin[6] = int8z_1[6];
    int16z_bin[7] = int8z_1[7];
    int16z_bin[8] = int8z_2[0];
    int16z_bin[9] = int8z_2[1];
    int16z_bin[10] = int8z_2[2];
    int16z_bin[11] = int8z_2[3];
    int16z_bin[12] = int8z_2[4];
    int16z_bin[13] = int8z_2[5]
    int16z_bin[14] = int8z_2[6];
    int16z_bin[15] = int8z_2[7];
  x0 -> Daten_einlesen
  (default) -> x0
  Daten_einlesen -> x1_1
  x1_1 -> Daten_einlesen
  data: int8z_1 input size=8; int8z_2 input size=8; int16z_bin output size=16 =0

== stateflow chart mobil_transporter/Modul Positionswerte Sampletime = 0.01 s/Chart2 ==
  state Daten_einlesen
  state x0
  state x1_1
    int16y_bin[0] = int8y_1[0];
    int16y_bin[1] = int8y_1[1];
    int16y_bin[2] = int8y_1[2];
    int16y_bin[3] = int8y_1[3];
    int16y_bin[4] = int8y_1[4];
    int16y_bin[5] = int8y_1[5]
    int16y_bin[6] = int8y_1[6];
    int16y_bin[7] = int8y_1[7];
    int16y_bin[8] = int8y_2[0];
    int16y_bin[9] = int8y_2[1];
    int16y_bin[10] = int8y_2[2];
    int16y_bin[11] = int8y_2[3];
    int16y_bin[12] = int8y_2[4];
    int16y_bin[13] = int8y_2[5]
    int16y_bin[14] = int8y_2[6];
    int16y_bin[15] = int8y_2[7];
  x0 -> Daten_einlesen
  (default) -> x0
  Daten_einlesen -> x1_1
  x1_1 -> Daten_einlesen
  data: int8y_1 input size=8; int8y_2 input size=8; int16y_bin output size=16 =0

== stateflow chart mobil_transporter/Uebergeben ==
  settings: sampleTime=0.001
  state unterfahren
    en:PWM=100;
    en:Richtung=0;
  state Wait
    en: give_fertig=1;
    en: PWM=0;
    en:Richtung=0;
  state Start
    en: PWM=0;
  state Pause
    en:give_fertig=0;
  state Hochfahren_2
    en:PWM=100;
    en:Richtung=1;
  state Give_fertig
    en:give_fertig=0;
  state Hochfahren_1
    en:PWM=100;
    en:Richtung=1;
  state Stop_and_Give_1
    en:PWM=0;
    en:Richtung=0;
  state Rueckfahren
    en:PWM=100;
    en:Richtung=0;
  state Stop_and_Give_2
    en:PWM=0;
    en:Richtung=1;
  state wait_to_start
    en:give_fertig=1;
  (default) -> unterfahren
  unterfahren -> Start : [UnterTaster_dif>0]
  Wait -> Pause : after(2,sec)
  Pause -> Hochfahren_2 : [start_ubergabe==1]
  Start -> Hochfahren_1 : [start_ubergabe==1]
  Rueckfahren -> Wait : [UnterTaster_dif>0]
  Hochfahren_2 -> Stop_and_Give_2 : [OberTaster==1]
  wait_to_start -> Give_fertig : after(2,sec)
  Hochfahren_1 -> Stop_and_Give_1 : [OberTaster==1]
  Stop_and_Give_1 -> Rueckfahren : after(5,sec)
  Stop_and_Give_2 -> wait_to_start : after(3,sec)
  data: OberTaster input double; UnterTaster_dif input double; PWM output double; Richtung output double; give_fertig output double; start_ubergabe input double

== stateflow chart mobil_transporter/Modul Positionswerte Sampletime = 0.01 s/Chart4 ==
  state Daten_einlesen
  state x0
  state x1_1
    int16a1_bin[0] = int8a1_1[0];
    int16a1_bin[1] = int8a1_1[1];
    int16a1_bin[2] = int8a1_1[2];
    int16a1_bin[3] = int8a1_1[3];
    int16a1_bin[4] = int8a1_1[4];
    int16a1_bin[5] = int8a1_1[5]
    int16a1_bin[6] = int8a1_1[6];
    int16a1_bin[7] = int8a1_1[7];
    int16a1_bin[8] = int8a1_2[0];
    int16a1_bin[9] = int8a1_2[1];
    int16a1_bin[10] = int8a1_2[2];
    int16a1_bin[11] = int8a1_2[3];
    int16a1_bin[12] = int8a1_2[4];
    int16a1_bin[13] = int8a1_2[5]
    int16a1_bin[14] = int8a1_2[6];
    int16a1_bin[15] = int8a1_2[7];
  x0 -> Daten_einlesen
  (default) -> x0
  Daten_einlesen -> x1_1
  x1_1 -> Daten_einlesen
  data: int8a1_1 input size=8; int8a1_2 input size=8; int16a1_bin output size=16 =0

== stateflow chart mobil_transporter/Modul Positionswerte Sampletime = 0.01 s/Chart6 ==
  state Daten_einlesen
  state x0
  state x1_1
    int16x_bin[0] = int8x_1[0];
    int16x_bin[1] = int8x_1[1];
    int16x_bin[2] = int8x_1[2];
    int16x_bin[3] = int8x_1[3];
    int16x_bin[4] = int8x_1[4];
    int16x_bin[5] = int8x_1[5]
    int16x_bin[6] = int8x_1[6];
    int16x_bin[7] = int8x_1[7];
    int16x_bin[8] = int8x_2[0];
    int16x_bin[9] = int8x_2[1];
    int16x_bin[10] = int8x_2[2];
    int16x_bin[11] = int8x_2[3];
    int16x_bin[12] = int8x_2[4];
    int16x_bin[13] = int8x_2[5]
    int16x_bin[14] = int8x_2[6];
    int16x_bin[15] = int8x_2[7];
  x0 -> Daten_einlesen
  (default) -> x0
  Daten_einlesen -> x1_1
  x1_1 -> Daten_einlesen
  data: int8x_1 input size=8; int8x_2 input size=8; int16x_bin output size=16 =0

== matlab function mobil_transporter/Navigation/Differenz von Winkel und Distanz/Restart Kontroller ==
  data: delta_D input; restart output
function restart = fcn(delta_D)
if  delta_D < 1000
    %% der Fahrzeug ist naehe vom Ziel
    restart = 1;
else
    restart = 0;
end

== matlab function mobil_transporter/Navigation/Differenz von Winkel und Distanz/alpha Soll Werte im Nexoner Koordinaten umrechnen ==
  settings: updateMethod=DISCRETE  sampleTime=0.01
  data: delta_x input; alpha_soll output; delta_y input
function alpha_soll = fcn( delta_x,delta_y)

if delta_y>0
    alpha_soll = atan2(delta_y,delta_x)*1800/pi;
else
    alpha_soll = atan2(delta_y,delta_x)*1800/pi+3600;
end

== matlab function mobil_transporter/Navigation/Distanz: Stufige PWM/Stufige PWM  ==
  data: delta_D input; y output
function y = fcn(delta_D)

if delta_D< 300
    %% anhalten
    y = 0;
else
    %% gerade fahren
    y = 90;

end

== matlab function mobil_transporter/Navigation/P Regler: Linear PWM/PWM_Minimum_Kontrollen Falls der Fahrzeug zu schwer ist, kann es sich nicht mehr bewegen.  ==
  data: u input; y output
function y = fcn(u)
if u<60
    %% Minimum des PWM
    y=60;
else
    y=u;
end

== matlab function mobil_transporter/Navigation/P Regler: Linear PWM/delta_alpha zur 180 Grad umrechnen damit es mit P Regler verknüpfen ==
  data: u input; y output
function y = fcn(u)
if 180 < u && u <350
    y = u-180;
elseif -350 < u && u < -180
    y = u + 180;
else
    y=u;
end
